simulink model "sampleModel2026"  (R2023a)
settings: Solver=VariableStepAuto  StartTime=0.0  StopTime=10.0  RelTol=1e-3
libraries: simulink x1, hdlsllib x1
settings Model: Creator=user1  LastModifiedBy=user1

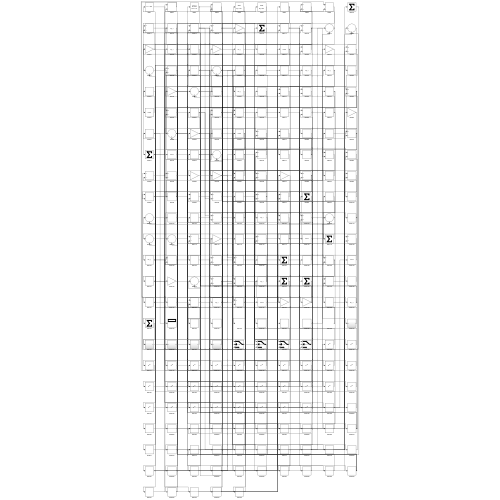
[thumbnail: Simulink's stored preview of the top-level diagram]
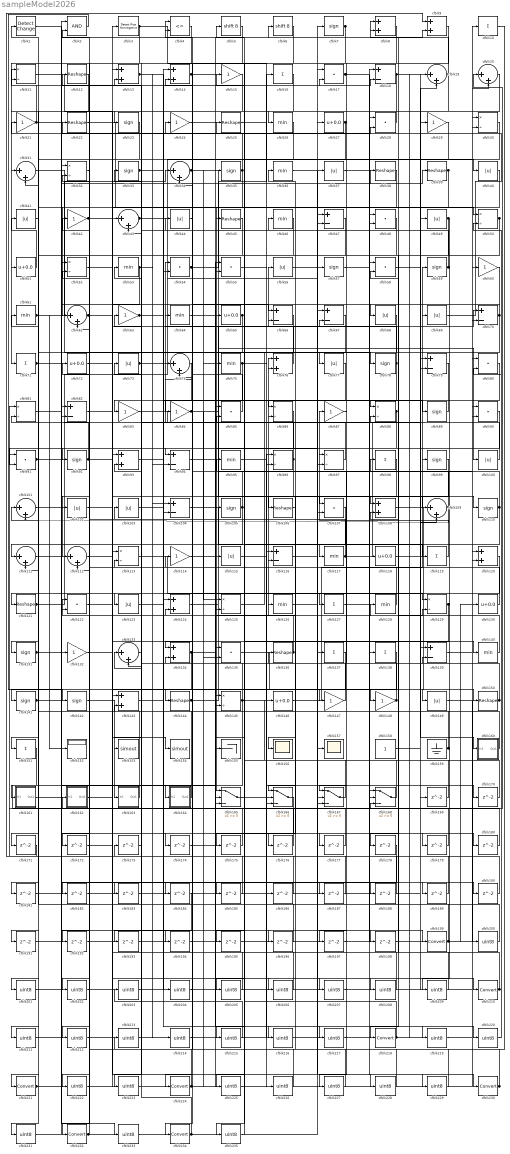
== system sampleModel2026 ==
  cfblk1 : simulink/Logic and Bit Operations/Detect Change  vinit=0  OutDataTypeStr=boolean
      settings: LibrarySourceBlock=|
      | hdlsllib/Logic and Bit
      | Operations/Detect
      | Change
  cfblk{10,16,71,98,119,127,137..138,151} (9 alike) : Sum  Inputs=+
  cfblk{37,40..41,44,49,56,68..69,73,77,100,102..103,115,123,149} (16 alike) : Abs  SaturateOnIntegerOverflow=off
  cfblk{19..20,31,34,43,62,74,101,109,111..112,133} (12 alike) : Sum  Inputs=|++
  cfblk{18,47,66..67,70,79,82,94,104,116,139} (11 alike) : Sum  Inputs=+-
  cfblk{7,23,33,35,57,59,78,89,92,99,105,110,131,141..142} (15 alike) : Signum
  cfblk{12,22,25,38..39,45,106,121,136,144,150} (11 alike) : Reshape
  cfblk{17,28,48,54..55,58,80,85,90..91,107,122,135} (13 alike) : DotProduct  OutDataTypeStr=Inherit: Inherit via internal rule
  cfblk{8..9,13..14,76,93,108,120,124,134,143} (11 alike) : Sum
  cfblk{11,30,32,50,52,81,86,88,96..97,113,125,129,145} (14 alike) : Product  Inputs=*/  RndMeth=Zero  SaturateOnIntegerOverflow=on
  cfblk{15,21,24,29,42,60,63,83..84,87,114,132,147..148} (14 alike) : Gain
  cfblk{26,36,46,53,61,64,75,95,117,126,128,140} (12 alike) : MinMax
  cfblk{27,51,65,72,118,130,146} (7 alike) : Bias  Bias=0.0  SaturateOnIntegerOverflow=off
  cfblk152 : Display
  cfblk153 : ToWorkspace  VariableName=simout  SaveFormat=Timeseries  SampleTime=-1
  cfblk154 : ToWorkspace  VariableName=simout  SaveFormat=Timeseries  SampleTime=-1
  cfblk155 : Terminator
  cfblk156 : Scope
  cfblk157 : Scope
  cfblk158 : Constant  SampleTime=-1
  cfblk159 : Ground
  cfblk160 : Subsystem
      settings: LibrarySourceBlock=|
      | hdlsllib/Ports &
      | Subsystems/Subsystem
  cfblk161 : Subsystem
      settings: LibrarySourceBlock=|
      | hdlsllib/Ports &
      | Subsystems/Subsystem
  cfblk162 : Subsystem
      settings: LibrarySourceBlock=|
      | hdlsllib/Ports &
      | Subsystems/Subsystem
  cfblk163 : Subsystem
      settings: LibrarySourceBlock=|
      | hdlsllib/Ports &
      | Subsystems/Subsystem
  cfblk164 : Subsystem
      settings: LibrarySourceBlock=|
      | hdlsllib/Ports &
      | Subsystems/Subsystem
  cfblk{165..168} (4 alike) : Switch  SaturateOnIntegerOverflow=off  InputSameDT=off
  cfblk{169..198} (30 alike) : Delay  SampleTime=1
  cfblk{199,210,218,221,224,230,232,234} (8 alike) : DataTypeConversion  SaturateOnIntegerOverflow=off  RndMeth=Floor
  cfblk2 : Logic  AllPortsSameDT=off  OutDataTypeStr=boolean
  cfblk{200..209,211..217,219..220,222..223,225..229,231,233,235} (29 alike) : DataTypeConversion  OutDataTypeStr=uint8  SaturateOnIntegerOverflow=off  RndMeth=Floor
  cfblk3 : hdlsllib/Logic and Bit Operations/Detect Rise Nonnegative  vinit=0  OutDataTypeStr=boolean
  cfblk4 : RelationalOperator  Operator=<=  OutDataTypeStr=boolean  InputSameDT=off
  cfblk5 : ArithShift  BitShiftNumber=8
  cfblk6 : ArithShift  BitShiftNumber=8
  wires:
  cfblk128/1 -> cfblk76/1
  cfblk125/1 -> cfblk78/1
  cfblk34/1 -> cfblk100/1, cfblk177/1
  cfblk137/1 -> cfblk232/1
  cfblk7/1 -> cfblk172/1, cfblk205/1
  cfblk28/1 -> cfblk26/1
  cfblk147/1 -> cfblk103/1
  cfblk130/1 -> cfblk72/1
  cfblk43/1 -> cfblk40/1, cfblk105/1
  cfblk53/1 -> cfblk104/1, cfblk94/2, cfblk82/2
  cfblk118/1 -> cfblk59/1
  cfblk91/1 -> cfblk38/1, cfblk196/1
  cfblk136/1 -> cfblk76/2, cfblk52/2
  cfblk69/1 -> cfblk25/1
  cfblk108/1 -> cfblk150/1
  cfblk47/1 -> cfblk221/1
  cfblk129/1 -> cfblk175/1, cfblk176/1
  cfblk124/1 -> cfblk67/2
  cfblk2/1 -> cfblk142/1
  cfblk77/1 -> cfblk164/1(In1)
  cfblk4/1 -> cfblk71/1
  cfblk22/1 -> cfblk165/1
  cfblk161/1(Out1) -> cfblk82/1
  cfblk119/1 -> cfblk87/1
  cfblk12/1 -> cfblk111/1
  cfblk64/1 -> cfblk106/1
  cfblk164/1(Out1) -> cfblk101/1
  cfblk148/1 -> cfblk53/1, cfblk97/1
  cfblk110/1 -> cfblk117/1, cfblk34/2
  cfblk92/1 -> cfblk61/1, cfblk107/1
  cfblk89/1 -> cfblk86/1
  cfblk151/1 -> cfblk20/1
  cfblk100/1 -> cfblk54/1
  cfblk146/1 -> cfblk99/1
  cfblk58/1 -> cfblk160/1(In1)
  cfblk103/1 -> cfblk54/2
  cfblk35/1 -> cfblk12/1, cfblk222/1
  cfblk135/1 -> cfblk149/1
  cfblk37/1 -> cfblk138/1
  cfblk133/1 -> cfblk33/1
  cfblk24/1 -> cfblk88/1
  cfblk78/1 -> cfblk56/1, cfblk36/1, cfblk107/2
  cfblk56/1 -> cfblk157/1
  cfblk50/1 -> cfblk52/1, cfblk192/1, cfblk193/1
  cfblk121/1 -> cfblk49/1, cfblk179/1
  cfblk18/1 -> cfblk79/1, cfblk182/1, cfblk225/1
  cfblk142/1 -> cfblk163/1(In1)
  cfblk158/1 -> cfblk139/1
  cfblk60/1 -> cfblk224/1
  cfblk99/1 -> cfblk156/1
  cfblk21/1 -> cfblk11/1, cfblk165/3
  cfblk16/1 -> cfblk23/1
  cfblk9/1 -> cfblk134/1
  cfblk45/1 -> cfblk104/2
  cfblk97/1 -> cfblk46/1
  cfblk80/1 -> cfblk218/1
  cfblk73/1 -> cfblk7/1, cfblk85/1
  cfblk167/1 -> cfblk146/1
  cfblk88/1 -> cfblk91/2, cfblk197/1
  cfblk117/1 -> cfblk29/1, cfblk62/2
  cfblk144/1 -> cfblk30/1, cfblk75/1
  cfblk105/1 -> cfblk44/1, cfblk111/2
  cfblk61/1 -> cfblk34/1, cfblk152/1
  cfblk48/1 -> cfblk144/1
  cfblk134/1 -> cfblk129/2, cfblk171/1, cfblk216/1
  cfblk15/1 -> cfblk51/1
  cfblk70/1 -> cfblk79/2, cfblk168/2, cfblk68/1
  cfblk51/1 -> cfblk41/1
  cfblk55/1 -> cfblk210/1
  cfblk31/1 -> cfblk118/1
  cfblk3/1 -> cfblk96/2, cfblk202/1
  cfblk106/1 -> cfblk166/1
  cfblk160/1(Out1) -> cfblk122/1
  cfblk96/1 -> cfblk135/1, cfblk13/2
  cfblk74/1 -> cfblk123/1
  cfblk168/1 -> cfblk15/1
  cfblk101/1 -> cfblk112/1
  cfblk67/1 -> cfblk74/2
  cfblk86/1 -> cfblk131/1
  cfblk145/1 -> cfblk4/1, cfblk167/3, cfblk191/1
  cfblk19/1 -> cfblk31/1, cfblk8/1
  cfblk68/1 -> cfblk166/2
  cfblk71/1 -> cfblk39/1, cfblk28/2, cfblk161/1(In1)
  cfblk54/1 -> cfblk16/1, cfblk129/1
  cfblk165/1 -> cfblk128/1
  cfblk132/1 -> cfblk230/1
  cfblk17/1 -> cfblk189/1, cfblk229/1
  cfblk140/1 -> cfblk98/1
  cfblk42/1 -> cfblk145/1, cfblk50/1, cfblk206/1
  cfblk85/1 -> cfblk21/1
  cfblk122/1 -> cfblk3/1
  cfblk29/1 -> cfblk45/1
  cfblk150/1 -> cfblk63/1, cfblk139/2
  cfblk79/1 -> cfblk153/1
  cfblk84/1 -> cfblk89/1, cfblk125/1
  cfblk26/1 -> cfblk166/3
  cfblk113/1 -> cfblk127/1
  cfblk114/1 -> cfblk65/1
  cfblk33/1 -> cfblk48/2, cfblk147/1
  cfblk66/1 -> cfblk151/1
  cfblk36/1 -> cfblk57/1
  cfblk104/1 -> cfblk119/1
  cfblk46/1 -> cfblk112/2
  cfblk131/1 -> cfblk32/1, cfblk233/1
  cfblk109/1 -> cfblk101/2, cfblk14/2
  cfblk14/1 -> cfblk9/2, cfblk97/2
  cfblk23/1 -> cfblk102/1
  cfblk13/1 -> cfblk108/1, cfblk214/1, cfblk217/1
  cfblk6/1 -> cfblk133/2
  cfblk59/1 -> cfblk109/1, cfblk11/2
  cfblk8/1 -> cfblk167/1
  cfblk107/1 -> cfblk155/1
  cfblk159/1 -> cfblk64/1, cfblk66/2
  cfblk81/1 -> cfblk6/1
  cfblk83/1 -> cfblk86/2
  cfblk11/1 -> cfblk113/1
  cfblk38/1 -> cfblk62/1
  cfblk65/1 -> cfblk165/2, cfblk125/2
  cfblk163/1(Out1) -> cfblk81/2
  cfblk20/1 -> cfblk83/1
  cfblk5/1 -> cfblk234/1
  cfblk76/1 -> cfblk24/1
  cfblk49/1 -> cfblk178/1, cfblk209/1
  cfblk112/1 -> cfblk69/1
  cfblk72/1 -> cfblk154/1
  cfblk62/1 -> cfblk66/1, cfblk140/1, cfblk17/2
  cfblk63/1 -> cfblk43/2, cfblk148/1, cfblk198/1
  cfblk139/1 -> cfblk20/2
  cfblk1/1 -> cfblk199/1
  cfblk141/1 -> cfblk18/2, cfblk181/1
  cfblk39/1 -> cfblk77/1, cfblk121/1
  cfblk75/1 -> cfblk84/1, cfblk167/2
  cfblk27/1 -> cfblk94/1, cfblk141/1
  cfblk57/1 -> cfblk110/1
  cfblk32/1 -> cfblk92/1
  cfblk127/1 -> cfblk70/1
  cfblk169/1 -> cfblk58/1
  cfblk25/1 -> cfblk170/1
  cfblk170/1 -> cfblk48/1
  cfblk171/1 -> cfblk9/1
  cfblk172/1 -> cfblk13/1
  cfblk173/1 -> cfblk133/1
  cfblk102/1 -> cfblk174/1
  cfblk175/1 -> cfblk81/1
  cfblk176/1 -> cfblk113/2
  cfblk177/1 -> cfblk31/2
  cfblk179/1 -> cfblk116/2
  cfblk94/1 -> cfblk180/1
  cfblk180/1 -> cfblk88/2
  cfblk181/1 -> cfblk145/2
  cfblk182/1 -> cfblk19/2
  cfblk40/1 -> cfblk183/1
  cfblk183/1 -> cfblk18/1
  cfblk44/1 -> cfblk184/1
  cfblk111/1 -> cfblk185/1
  cfblk185/1 -> cfblk2/1
  cfblk115/1 -> cfblk186/1
  cfblk186/1 -> cfblk122/2
  cfblk138/1 -> cfblk187/1
  cfblk187/1 -> cfblk14/1
  cfblk162/1(Out1) -> cfblk188/1
  cfblk188/1 -> cfblk28/1
  cfblk189/1 -> cfblk168/3
  cfblk82/1 -> cfblk190/1
  cfblk190/1 -> cfblk91/1
  cfblk191/1 -> cfblk109/2
  cfblk192/1 -> cfblk2/2
  cfblk193/1 -> cfblk96/1
  cfblk52/1 -> cfblk194/1
  cfblk194/1 -> cfblk30/2
  cfblk98/1 -> cfblk195/1
  cfblk195/1 -> cfblk168/1
  cfblk196/1 -> cfblk134/2
  cfblk197/1 -> cfblk70/2
  cfblk198/1 -> cfblk108/2
  cfblk199/1 -> cfblk8/2, cfblk130/1
  cfblk149/1 -> cfblk200/1
  cfblk200/1 -> cfblk1/1
  cfblk120/1 -> cfblk201/1
  cfblk201/1 -> cfblk124/1
  cfblk202/1 -> cfblk120/1
  cfblk203/1 -> cfblk120/2
  cfblk143/1 -> cfblk204/1
  cfblk204/1 -> cfblk74/1
  cfblk205/1 -> cfblk143/1
  cfblk206/1 -> cfblk143/2
  cfblk93/1 -> cfblk207/1
  cfblk207/1 -> cfblk169/1
  cfblk123/1 -> cfblk208/1
  cfblk208/1 -> cfblk93/1
  cfblk209/1 -> cfblk93/2
  cfblk210/1 -> cfblk50/2, cfblk114/1, cfblk58/2
  cfblk30/1 -> cfblk211/1
  cfblk211/1 -> cfblk55/1
  cfblk178/1 -> cfblk212/1
  cfblk212/1 -> cfblk55/2
  cfblk10/1 -> cfblk213/1
  cfblk213/1 -> cfblk116/1
  cfblk214/1 -> cfblk10/1
  cfblk90/1 -> cfblk215/1
  cfblk215/1 -> cfblk73/1
  cfblk216/1 -> cfblk90/1
  cfblk217/1 -> cfblk90/2
  cfblk218/1 -> cfblk85/2, cfblk19/1
  cfblk174/1 -> cfblk219/1
  cfblk219/1 -> cfblk80/1
  cfblk116/1 -> cfblk220/1
  cfblk220/1 -> cfblk80/2
  cfblk221/1 -> cfblk37/1, cfblk115/1, cfblk43/1
  cfblk222/1 -> cfblk47/1
  cfblk184/1 -> cfblk223/1
  cfblk223/1 -> cfblk47/2
  cfblk224/1 -> cfblk32/2, cfblk135/2, cfblk35/1
  cfblk225/1 -> cfblk60/1
  cfblk95/1 -> cfblk226/1
  cfblk226/1 -> cfblk22/1
  cfblk87/1 -> cfblk227/1
  cfblk227/1 -> cfblk95/1
  cfblk126/1 -> cfblk228/1
  cfblk228/1 -> cfblk162/1(In1)
  cfblk229/1 -> cfblk126/1
  cfblk230/1 -> cfblk173/1, cfblk124/2, cfblk4/2, cfblk136/1
  cfblk41/1 -> cfblk231/1
  cfblk231/1 -> cfblk132/1
  cfblk232/1 -> cfblk42/1, cfblk67/1
  cfblk233/1 -> cfblk137/1
  cfblk234/1 -> cfblk203/1, cfblk17/1, cfblk27/1
  cfblk166/1 -> cfblk235/1
  cfblk235/1 -> cfblk5/1

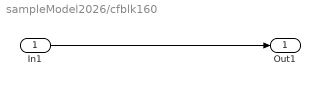
== system sampleModel2026/cfblk160 ==
  In1 : Inport
  Out1 : Outport
  wires:
  In1/1 -> Out1/1

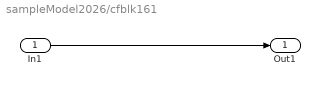
== system sampleModel2026/cfblk161 ==
  In1 : Inport
  Out1 : Outport
  wires:
  In1/1 -> Out1/1

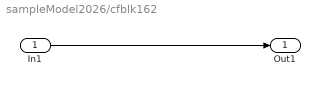
== system sampleModel2026/cfblk162 ==
  In1 : Inport
  Out1 : Outport
  wires:
  In1/1 -> Out1/1

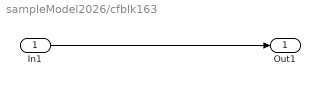
== system sampleModel2026/cfblk163 ==
  In1 : Inport
  Out1 : Outport
  wires:
  In1/1 -> Out1/1

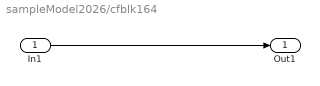
== system sampleModel2026/cfblk164 ==
  In1 : Inport
  Out1 : Outport
  wires:
  In1/1 -> Out1/1
